simulink model "EPS_loads"  (R2019b)
settings: Solver=VariableStepAuto  StartTime=0.0  StopTime=10.0  RelTol=1e-3
values from neighbouring files (symbols this model uses):
  eff_i1 = 0.9    [demoEPS.m]    (also in demoEPS_R2019a.m; demoEPS_v1.m; demoEPS_v1a.m; demoEPS_v1test.m)
  eff_i2 = 0.85    [demoEPS.m]    (also in demoEPS_R2019a.m; demoEPS_v1.m; demoEPS_v1a.m; demoEPS_v1test.m)
  Pload1 = 50    [demoEPS.m]    (also in demoEPS_R2019a.m; demoEPS_v1.m; demoEPS_v1a.m; demoEPS_v1test.m)
  Pload2 = 2    [demoEPS.m]    (also in demoEPS_R2019a.m; demoEPS_v1.m; demoEPS_v1a.m; demoEPS_v1test.m)
  Pload3 = 2.5    [demoEPS.m]    (also in demoEPS_R2019a.m; demoEPS_v1.m; demoEPS_v1a.m; demoEPS_v1test.m)
  Torbit = 2*pi*sqrt(((h+6378)^3)/398600)/60    [calc_mass_EPS.m]    (also in demoEPS.m = 5400; demoEPS_R2019a.m = 2*pi*sqrt(a^3/(3.986004418E5)); demoEPS_v1.m = 5400; demoEPS_v1a.m = 2*pi*sqrt(a^3/(3.986004418E5)))
libraries: simulink x1
settings Model: Creator=Ricardo  LastModifiedBy=Ricardo

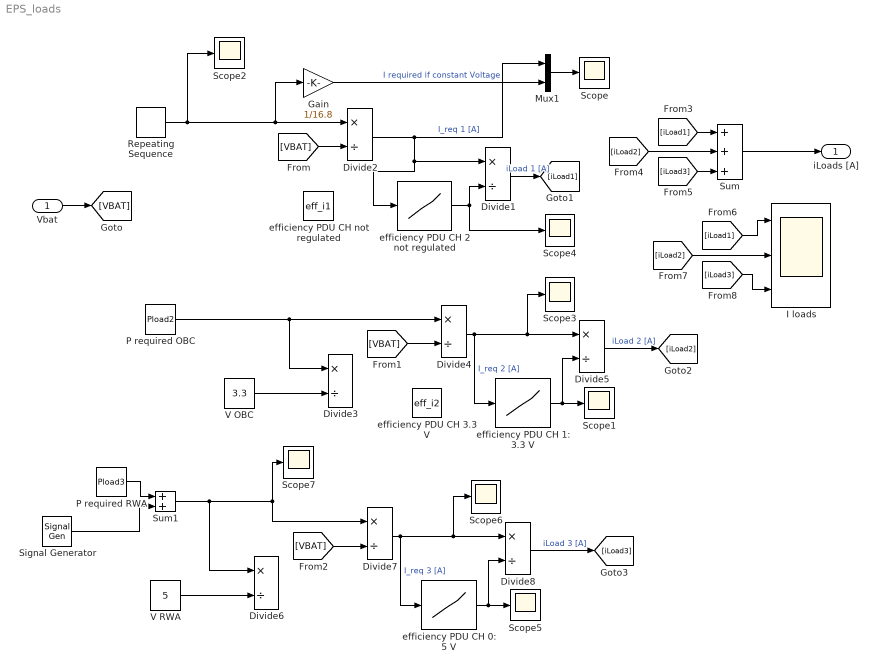
== system EPS_loads ==
  Vbat : Inport
  Divide{1..8} (8 alike) : Product  Inputs=*/
  Gain : Gain  Gain=1/16.8
  I loads : Scope  NumInputPorts=3
  Mux1 : Mux  Inputs=2
  P required OBC : Constant  Value=Pload2
  P required RWA : Constant  Value=Pload3
  Repeating Sequence : simulink/Sources/Repeating Sequence  rep_seq_t=[0, 1, (Torbit/2),(Torbit/2)+1, Torbit]  rep_seq_y=[0 Pload1 Pload1 0 0]
  Scope{,1..7} (8 alike) : Scope
  Signal Generator : SignalGenerator  WaveForm=random  Frequency=0.01
  Sum : Sum  Inputs=+++
  Sum1 : Sum
  V OBC : Constant  Value=3.3
  V RWA : Constant  Value=5
  efficiency PDU CH 0: 5 V : Lookup_n-D  NumberOfTableDimensions=1  BreakpointsForDimension1=[0,0.15,0.18,0.25,0.4,0.5,0.75,1,1.5,2]  Table=[0,0.65,0.7,0.8,0.85,0.88,0.89,0.9,0.88,0.87]  InternalRulePriority=Speed  RndMeth=Simplest  InputSameDT=on
  efficiency PDU CH 1: 3.3 V : Lookup_n-D  NumberOfTableDimensions=1  BreakpointsForDimension1=[0,0.15,0.18,0.25,0.4,0.5,0.75,1,1.5,2]  Table=[0,0.65,0.7,0.8,0.85,0.88,0.89,0.9,0.88,0.87]  InternalRulePriority=Speed  RndMeth=Simplest  InputSameDT=on
  efficiency PDU CH 2 not regulated : Lookup_n-D  NumberOfTableDimensions=1  BreakpointsForDimension1=[0,0.15,0.2,0.25,0.4,0.5,0.75,1,1.5,2]  Table=[0.25,0.97,0.99,0.98594,0.97572,0.96294,0.95783,0.95783,0.94505,0.93994]  InternalRulePriority=Speed  RndMeth=Simplest  InputSameDT=on
  efficiency PDU CH 3.3 V : Constant  Value=eff_i2
  efficiency PDU CH not regulated : Constant  Value=eff_i1
  iLoads [A] : Outport
  wires:
  Sum/1 -> iLoads [A]/1
  P required OBC/1 -> Divide4/1, Divide3/1
  Repeating Sequence/1 -> Scope2/1, Gain/1, Divide2/1
  P required RWA/1 -> Sum1/1
  efficiency PDU CH 2 not regulated/1 -> Scope4/1, Divide1/2
  V OBC/1 -> Divide3/2
  Divide4/1 -> efficiency PDU CH 1: 3.3 V/1, Scope3/1, Divide5/1  "I_req 2 [A]"
  efficiency PDU CH 1: 3.3 V/1 -> Scope1/1, Divide5/2
  Divide2/1 -> Mux1/1, efficiency PDU CH 2 not regulated/1, Divide1/1  "I_req 1 [A]"
  [VBAT] -> Divide4/2
  Signal Generator/1 -> Sum1/2
  Sum1/1 -> Divide6/1, Divide7/1, Scope7/1
  Divide5/1 -> [iLoad2]  "iLoad 2 [A]"
  Vbat/1 -> [VBAT]
  Divide1/1 -> [iLoad1]  "iLoad 1 [A]"
  [iLoad3] -> I loads/3
  [iLoad1] -> Sum/1
  [iLoad2] -> Sum/2
  [iLoad3] -> Sum/3
  [iLoad2] -> I loads/2
  Divide7/1 -> efficiency PDU CH 0: 5 V/1, Scope6/1, Divide8/1  "I_req 3 [A]"
  Gain/1 -> Mux1/2  "I required if constant Voltage"
  efficiency PDU CH 0: 5 V/1 -> Scope5/1, Divide8/2
  [VBAT] -> Divide7/2
  [iLoad1] -> I loads/1
  Mux1/1 -> Scope/1
  [VBAT] -> Divide2/2
  V RWA/1 -> Divide6/2
  Divide8/1 -> [iLoad3]  "iLoad 3 [A]"
